simulink library "CommonLib"  (R2024b)
settings: Solver=VariableStepAuto  StartTime=0.0  StopTime=10.0  RelTol=1e-3
settings Model: Creator=sunha  LastModifiedBy=sunha

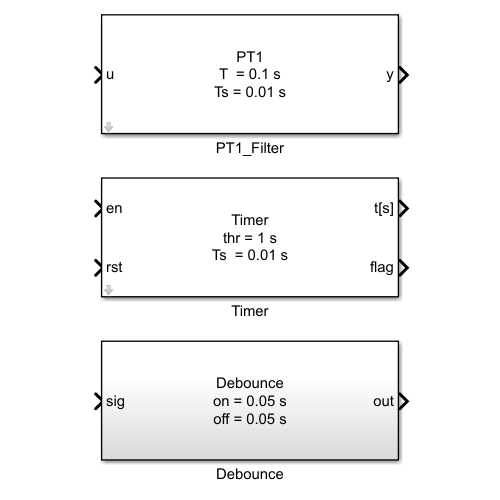
[thumbnail: Simulink's stored preview of the top-level diagram]
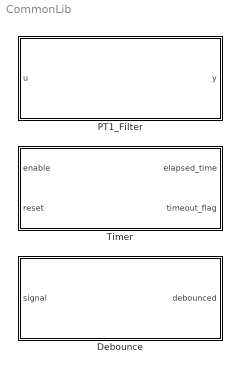
== system CommonLib ==
  Debounce : Subsystem  mask{Ts=0.01, on_delay=0.05, off_delay=0.05}
      mask prompts: Ts "샘플타임 Ts [s]"; on_delay "ON 확정 딜레이 [s]"; off_delay "OFF 확정 딜레이 [s]"
      mask help:
      | Debounce: 노이즈성 신호를 안정화합니다.
      |
      |   signal이 on_delay [s] 이상 연속 1  → 출력 1
      |   signal이 off_delay [s] 이상 연속 0 → 출력 0
      |   그 외 → 이전 값 유지
      |
      | on_delay = off_delay 로 설정하면 대칭 디바운스
      mask Display:
      | port_label('input',  1, 'sig')
      | port_label('output', 1, 'out')
      | disp(sprintf('Debounce\non = %g s\noff = %g s', on_delay, off_delay))
  PT1_Filter : Subsystem  mask{T=0.1, Ts=0.01}
      mask prompts: T "시정수 T [s]"; Ts "샘플타임 Ts [s]"
      mask help:
      | PT1 1차 저역통과 필터 (Forward Euler 이산화)
      |
      | y[k] = (1 - Ts/T)*y[k-1] + (Ts/T)*u[k]
      |
      |   T  : 시정수 (클수록 느리게 반응)
      |   Ts : 샘플타임 (상위 모델과 일치시킬 것)
      mask Display:
      | port_label('input',  1, 'u')
      | port_label('output', 1, 'y')
      | disp(sprintf('PT1\nT  = %g s\nTs = %g s', T, Ts))
  Timer : Subsystem  mask{Ts=0.01, threshold=1.0}
      mask prompts: Ts "샘플타임 Ts [s]"; threshold "타임아웃 기준 threshold [s]"
      mask help:
      | Timer: enable=1 동안 경과시간을 카운트합니다.
      |
      |   reset=1  → 즉시 0으로 초기화 (최우선)
      |   enable=1 → 매 스텝 Ts씩 증가
      |   enable=0 → 현재값 유지
      |
      |   timeout_flag = elapsed_time >= threshold
      mask Display:
      | port_label('input',  1, 'en')
      | port_label('input',  2, 'rst')
      | port_label('output', 1, 't[s]')
      | port_label('output', 2, 'flag')
      | disp(sprintf('Timer\nthr = %g s\nTs  = %g s', threshold, Ts))

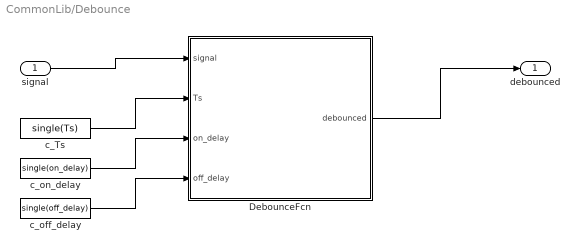
== system CommonLib/Debounce ==
  signal : Inport
  DebounceFcn : MATLAB Function  TreatAsAtomicUnit=on
  c_Ts : Constant  Value=single(Ts)  OutDataTypeStr=single
  c_off_delay : Constant  Value=single(off_delay)  OutDataTypeStr=single
  c_on_delay : Constant  Value=single(on_delay)  OutDataTypeStr=single
  debounced : Outport
  wires:
  signal/1 -> DebounceFcn/1(signal)
  c_Ts/1 -> DebounceFcn/2(Ts)
  c_on_delay/1 -> DebounceFcn/3(on_delay)
  c_off_delay/1 -> DebounceFcn/4(off_delay)
  DebounceFcn/1(debounced) -> debounced/1

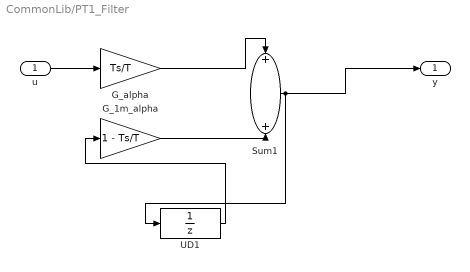
== system CommonLib/PT1_Filter ==
  u : Inport  OutDataTypeStr=single
  G_1m_alpha : Gain  Gain=1 - Ts/T  OutDataTypeStr=single
  G_alpha : Gain  Gain=Ts/T  OutDataTypeStr=single
  Sum1 : Sum
  UD1 : UnitDelay  InitialCondition=single(0)
  y : Outport
  wires:
  u/1 -> G_alpha/1
  G_alpha/1 -> Sum1/1
  UD1/1 -> G_1m_alpha/1
  G_1m_alpha/1 -> Sum1/2
  Sum1/1 -> y/1, UD1/1

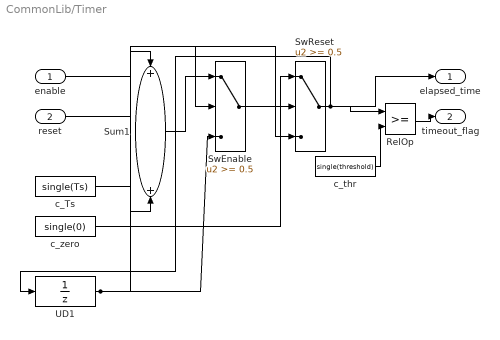
== system CommonLib/Timer ==
  enable : Inport
  reset : Inport  Port=2
  RelOp : RelationalOperator
  Sum1 : Sum
  SwEnable : Switch  Threshold=0.5
  SwReset : Switch  Threshold=0.5
  UD1 : UnitDelay  InitialCondition=single(0)
  c_Ts : Constant  Value=single(Ts)  OutDataTypeStr=single
  c_thr : Constant  Value=single(threshold)  OutDataTypeStr=single
  c_zero : Constant  Value=single(0)  OutDataTypeStr=single
  elapsed_time : Outport
  timeout_flag : Outport  Port=2
  wires:
  UD1/1 -> Sum1/1, SwEnable/3
  c_Ts/1 -> Sum1/2
  Sum1/1 -> SwEnable/1
  enable/1 -> SwEnable/2
  c_zero/1 -> SwReset/1
  reset/1 -> SwReset/2
  SwEnable/1 -> SwReset/3
  SwReset/1 -> elapsed_time/1, UD1/1, RelOp/1
  c_thr/1 -> RelOp/2
  RelOp/1 -> timeout_flag/1

== matlab function CommonLib/Debounce/DebounceFcn ==
  data: signal input; debounced output; Ts input; on_delay input; off_delay input
function debounced = fcn(signal, Ts, on_delay, off_delay)
